simulink model "Refined_Model_42"  (R2020b)
settings: Solver=FixedStepAuto  StartTime=0.0  StopTime=300  FixedStep=dt  RelTol=1e-3
values from neighbouring files (symbols this model uses):
  ALInpSpeed = AxlLoss (1,:)    [GPS_val.m]    (also in ICEBEV_Script.m; ICEBEV_Script_VECTO.m; ICE_Script.m; ICE_Script_SSVal.m)
  ALInpTor = AxlLoss(:,1)    [GPS_val.m]    (also in ICEBEV_Script.m; ICEBEV_Script_VECTO.m; ICE_Script.m; ICE_Script_SSVal.m)
  ALTableVal = AxlLoss(2:end,2:end)    [GPS_val.m]    (also in ICEBEV_Script.m; ICEBEV_Script_VECTO.m; ICE_Script.m; ICE_Script_SSVal.m)
  CovDist = RoadProfile(:,4)    [ICE_Val.m]
  Cx = VehicleDefine(7,3)    [BEV_Basictest.m]    (also in GPS_val.m; ICEBEV_Script.m; ICEBEV_Script_VECTO.m; ICE_Script.m)
  Dist = 1:length(MaxSpeedProfile)    [GPS_val.m]    (also in ICE_Script.m; ICE_Val.m = [1:CovDist(end)])
  DynRolRad = VehicleDefine(5,3)    [BEV_Basictest.m]    (also in GPS_val.m; ICEBEV_Script.m; ICEBEV_Script_VECTO.m; ICE_Script.m)
  EngineRpm = round(IntpTorCur(:,1))    [GPS_val.m]    (also in ICEBEV_Script.m; ICEBEV_Script_VECTO.m; ICE_Script.m; ICE_Script_SSVal.m)
  EngineRpmRaw = TorCurRaw(:,1)    [GPS_val.m]    (also in ICEBEV_Script.m; ICEBEV_Script_VECTO.m; ICE_Script.m; ICE_Script_SSVal.m)
  EngineRpmUse = [EngineRpmUse1; EngineRpmUse2]    [GPS_val.m]    (also in ICEBEV_Script.m; ICEBEV_Script_VECTO.m; ICE_Script.m; ICE_Script_SSVal.m)
  etaClutch = VehicleDefine(23,3)    [GPS_val.m]    (also in ICEBEV_Script.m; ICEBEV_Script_VECTO.m; ICE_Script.m; ICE_Script_SSVal.m)
  FCTableVal = FCMap(2:end,2:end)    [GPS_val.m]    (also in ICEBEV_Script.m; ICEBEV_Script_VECTO.m; ICE_Script.m; ICE_Script_SSVal.m)
  FDR = VehicleDefine(20,3)    [BEV_Basictest.m]    (also in GPS_val.m = VehicleDefine(22,3); ICEBEV_Script.m = VehicleDefine(22,3); ICEBEV_Script_VECTO.m = VehicleDefine(22,3); ICE_Script.m = VehicleDefine(22,3))
  Fr = VehicleDefine(13,3)    [BEV_Basictest.m]    (also in GPS_val.m; ICEBEV_Script.m; ICEBEV_Script_VECTO.m; ICE_Script.m)
  g = VehicleDefine(14,3)    [BEV_Basictest.m]    (also in GPS_val.m; ICEBEV_Script.m; ICEBEV_Script_VECTO.m; ICE_Script.m)
  GNo = GBXDefine(:,1)    [GPS_val.m]    (also in ICEBEV_Script.m; ICEBEV_Script_VECTO.m; ICE_Script.m; ICE_Script_SSVal.m)
  GRa = GBXDefine(:,2)    [GPS_val.m]    (also in ICEBEV_Script.m; ICEBEV_Script_VECTO.m; ICE_Script.m; ICE_Script_SSVal.m)
  InitVel = VehicleDefine(21,3)    [BEV_Basictest.m]    (also in GPS_val.m = VehicleDefine(24,3); ICEBEV_Script.m = VehicleDefine(24,3); ICEBEV_Script_VECTO.m = VehicleDefine(24,3); ICE_Script.m = VehicleDefine(24,3))
  IntpSlope = round(IntpSlope,1)    [GPS_val.m]    (also in ICE_Script.m; ICE_Val.m = A)
  Je = VehicleDefine(25,3)    [GPS_val.m]    (also in ICEBEV_Script.m; ICEBEV_Script_VECTO.m; ICE_Script.m; ICE_Script_SSVal.m)
  Jk = VehicleDefine(15,3)    [BEV_Basictest.m]    (also in GPS_val.m; ICEBEV_Script.m; ICEBEV_Script_VECTO.m; ICE_Script.m)
  Jm = VehicleDefine(16,3)    [GPS_val.m]    (also in ICEBEV_Script.m; ICEBEV_Script_VECTO.m; ICE_Script.m; ICE_Script_SSVal.m)
  MaxAcc = 1    [BEV_Basictest.m]    (also in GPS_val.m; ICEBEV_Script.m; ICEBEV_Script_VECTO.m; ICE_Script.m)
  MaxDec = 1    [BEV_Basictest.m]    (also in GPS_val.m; ICEBEV_Script.m; ICEBEV_Script_VECTO.m; ICE_Script.m)
  MaxSpeedProfile = FMSP    [GPS_val.m]    (also in ICE_Script.m; ICE_Val.m = repelem(SegSPLatinmps,SegLeninm))
  MaxTorValThrot = max(ThrotTableVal,[],2)    [GPS_val.m]    (also in ICEBEV_Script.m; ICEBEV_Script_VECTO.m; ICE_Script.m; ICE_Script_SSVal.m)
  Me = VehicleDefine(10,3)    [BEV_Basictest.m]    (also in GPS_val.m; ICEBEV_Script.m; ICEBEV_Script_VECTO.m; ICE_Script.m)
  MotoringTor = IntpTorCur(:,3)    [GPS_val.m]    (also in ICEBEV_Script.m; ICEBEV_Script_VECTO.m; ICE_Script.m; ICE_Script_SSVal.m)
  Mt = VehicleDefine(12,3)    [BEV_Basictest.m]    (also in GPS_val.m; ICEBEV_Script.m; ICEBEV_Script_VECTO.m; ICE_Script.m)
  Mtot = Mv+Me+Mt    [BEV_Basictest.m]    (also in GPS_val.m; ICEBEV_Script.m; ICEBEV_Script_VECTO.m; ICE_Script.m)
  Mv = VehicleDefine(9,3)    [BEV_Basictest.m]    (also in GPS_val.m; ICEBEV_Script.m; ICEBEV_Script_VECTO.m; ICE_Script.m)
  NoSteps = round(Dist(end))    [GPS_val.m]    (also in ICE_Script.m; ICE_Val.m = 3002)
  NoWhlFA = VehicleDefine(2,3)    [BEV_Basictest.m]    (also in GPS_val.m; ICE_Script.m; ICE_Val.m; ICE_Val_new.m)
  NoWhlRA = VehicleDefine(4,3)    [BEV_Basictest.m]    (also in GPS_val.m; ICE_Script.m; ICE_Val.m; ICE_Val_new.m)
  rho = VehicleDefine(6,3)    [BEV_Basictest.m]    (also in GPS_val.m; ICEBEV_Script.m; ICEBEV_Script_VECTO.m; ICE_Script.m)
  RpmBrkPnt = ThrottleMap(1,:)    [GPS_val.m]    (also in ICEBEV_Script.m; ICEBEV_Script_VECTO.m; ICE_Script.m; ICE_Script_SSVal.m)
  s = divisors(length(MaxSpeedProfile))    [GPS_val.m]    (also in ICEBEV_Script.m = round(FLoadTor); ICEBEV_Script_VECTO.m = round(FLoadTor); ICE_Script.m = round(FLoadTor); ICE_Script_SSVal.m = round(FLoadTor))
  SegNo = RoadProfile(:,1)    [ICE_Val.m]
  SegSPLatinmps = (sqrt(aMaxLat*g*CurRadinm))    [GPS_val.m]    (also in ICE_Script.m; ICE_Val.m)
  Sx = VehicleDefine(8,3)    [BEV_Basictest.m]    (also in GPS_val.m; ICEBEV_Script.m; ICEBEV_Script_VECTO.m; ICE_Script.m)
  ThrotPos = ThrotPos'    [GPS_val.m]    (also in ICEBEV_Script.m; ICEBEV_Script_VECTO.m; ICE_Script.m; ICE_Script_SSVal.m)
  ThrotTableVal = ThrottleMap(2:end,2:end)    [GPS_val.m]    (also in ICEBEV_Script.m; ICEBEV_Script_VECTO.m; ICE_Script.m; ICE_Script_SSVal.m)
undefined symbols (not defined in the file or in its folder): G1Inprpm, GInprpm, GInpTor, Gmot, GTorLoss, Jgbx, MaxSpinG, MaxWhlTorinG, Stoptimes
libraries: simulink x3, autolibdatasheetbattery x1, autolibmappedmotor x1, autolibshared x1
(part 2 of 2)

== system Refined_Model_42/Driver Model/Gear and Clutch Definition/Clutch position definition/If Action Subsystem4 ==
  CL : Inport
  Action Port : ActionPort  ActionPortLabel=else
  CLO : Outport
  wires:
  CL/1 -> CLO/1

== system Refined_Model_42/Driver Model/Gear and Clutch Definition/Clutch position definition/Triggered Single Pulse ==
  Trigger : Inport
  +ve edge detect : Subsystem
  Add : Sum
  Add1 : Sum
  Compare To Constant : simulink/Logic and Bit Operations/Compare To Constant  relop=>  const=p_wid-1  OutDataTypeStr=boolean
  Constant2 : Constant
  Logical Operator : Logic  Operator=NOT  AllPortsSameDT=off  OutDataTypeStr=boolean
  Product : Product  RndMeth=Zero
  Product1 : Product  RndMeth=Zero
  Product3 : Product  RndMeth=Zero
  Saturation : Saturate  UpperLimit=1  LowerLimit=0
  Unit Delay : UnitDelay  SampleTime=-1  HasFrameUpgradeWarning=on
  Unit Delay1 : UnitDelay  SampleTime=-1  HasFrameUpgradeWarning=on
  Pulse : Outport
  wires:
  Compare To Constant/1 -> Logical Operator/1
  Constant2/1 -> Product/1
  Product/1 -> Add/1
  Unit Delay/1 -> Add/2, Compare To Constant/1
  Trigger/1 -> +ve edge detect/1(signal)
  +ve edge detect/1(out) -> Add1/2
  Add/1 -> Product1/2
  Product1/1 -> Unit Delay/1
  Add1/1 -> Unit Delay1/1
  Unit Delay1/1 -> Saturation/1
  Saturation/1 -> Product3/1
  Product3/1 -> Add1/1, Product/2, Product1/1, Pulse/1
  Logical Operator/1 -> Product3/2

== system Refined_Model_42/Driver Model/Gear and Clutch Definition/Clutch position definition/Triggered Single Pulse/+ve edge detect ==
  note: Edge
  signal : Inport
  Delay Input1 : UnitDelay  Description=Store in Global RAM  DisableCoverage=on  SampleTime=-1  HasFrameUpgradeWarning=on
  FixPt Relational Operator : RelationalOperator  Operator=>  OutDataTypeStr=fixdt(0, 8)  ZeroCross=off  RndMeth=Nearest
  Positive : simulink/Logic and Bit Operations/Compare To Zero  relop=>  OutDataTypeStr=uint8  ZeroCross=off
  out : Outport
  wires:
  Delay Input1/1 -> FixPt Relational Operator/2  "U(k-1)"
  Positive/1 -> Delay Input1/1, FixPt Relational Operator/1  "U(k)"
  FixPt Relational Operator/1 -> out/1
  signal/1 -> Positive/1

== stateflow chart Refined_Model_42/Driver Model/Acc//Dec Control/Driving State ==
  state Driving
    idle = 0;
    Bor = 0;
    Aor = 1;
    error = 0;
  state Stopping
    idle = 0;
    Bor = 1;
    Aor = 0;
    error = 0;
  state Calibration
    idle = 1;
    Bor = 0;
    Aor = 0;
    error = Dist2Stop;
  state Idling
    idle = 1;
    Bor = 0;
    Aor = 0;
    error = 0;
  (default) -> Driving
  Driving -> Stopping : [Dist2Stop <= Dist2Dec && UpSp < v]
  Calibration -> Driving : after(Stoptime - 1,sec) [v == 0 && a == 0]
  Stopping -> Idling : [v == 0 && d > 0 && Dist2Stop <= 1]
  Idling -> Calibration : after(1,sec)[Dist2Stop <= 1]{idle = 1}
  data: v input; a input; d input; idle output =0; Bor output; Stoptime input; Dist2Stop input; Dist2Dec input; UpSp input; error output; Aor output
